simulink model "LKAS"  (R2023b)
settings: Solver=FixedStepDiscrete  StartTime=0.0  StopTime=50  RelTol=1e-3  EnableMultiTasking=on
undefined symbols (not defined in the file): Rec, SDTV
libraries: visionconversions x2, visiongeotforms x2, dspvision x1, slpidlib x1
settings Model: Creator=Aral_Sarrafi  LastModifiedBy=seame-workstation09
settings SolverCC: AlgebraicLoopSolver=TrustRegion  PositivePriorityOrder=on
settings DataIOCC: ReturnWorkspaceOutputs=off
settings OptimizationCC: UseDivisionForNetSlopeComputation=on  GainParamInheritBuiltInType=on  UseFloatMulNetSlope=on  PassReuseOutputArgsAs=Individual arguments  ZeroExternalMemoryAtStartup=off  ZeroInternalMemoryAtStartup=off  NoFixptDivByZeroProtection=on  EfficientFloat2IntCast=on  LifeSpan=1  MaxStackSize=64  OptimizeBlockOrder=speed  OptimizationPriority=Speed  LabelGuidedReuse=on  MultiThreadedLoops=on  EfficientTunableParamExpr=on
settings DebuggingCC: ParameterTunabilityLossMsg=error  UnconnectedInputMsg=warning  UnconnectedOutputMsg=warning  UnconnectedLineMsg=warning  ArithmeticOperatorsInVariantConditions=warning
settings HardwareCC: ProdBitPerPointer=32  ProdBitPerSizeT=32  ProdBitPerPtrDiffT=32  ProdLargestAtomicInteger=Long  ProdLargestAtomicFloat=Double  ProdWordSize=32  ProdLongLongMode=on  ProdHWDeviceType=ARM Compatible->ARM Cortex  TargetBitPerLong=64  TargetBitPerPointer=64  TargetBitPerSizeT=64  TargetBitPerPtrDiffT=64  TargetLongLongMode=on  TargetIntDivRoundTo=Zero  TargetEndianess=LittleEndian  TargetWordSize=64  TargetHWDeviceType=MATLAB Host  ProdEqTarget=off
settings ModelReferenceCC: EnableRefExpFcnMdlSchedulingChecks=on
settings SFSimCC: SimUseLocalCustomCode=off  SimGenImportedTypeDefs=on  MATLABDynamicMemAllocThreshold=0  CustomCodeUndefinedFunction=UseInterfaceOnly  SimTargetLang=C++
settings RTWCC: Description=Embedded Coder  SystemTargetFile=ert.tlc  HardwareBoard=Raspberry Pi  TLCOptions="-aInlineSetEventsForThisBaseRateFcn=TLC_TRUE -aSuppressMultiTaskScheduler=TLC_FALSE  -aRateBasedStepFcn=0"  PackageGeneratedCodeAndArtifacts=on  TemplateMakefile=ert_default_tmf  RTWUseLocalCustomCode=off  TargetLang=C++
settings CodeAppCC: ForceParamTrailComments=on  IgnoreCustomStorageClasses=off  MaxIdLength=63  OperatorAnnotations=on  SimulinkDataObjDesc=on  SFDataObjDesc=on  CustomSymbolStrGlobalVar=rt$N$M  CustomSymbolStrType=$N$M  CustomSymbolStrFcn=$N$M$F  CustomSymbolStrMacro=$N$M  InsertBlockDesc=on
settings ERTTargetCC: IncludeMdlTerminateFcn=off  CombineSignalStateStructs=on  SupportAbsoluteTime=off  SupportComplex=off  SupportNonInlinedSFcns=on  SupportVariableSizeSignals=on  OptimizeReductions=on  ExtModeTransport=2  ExtModeStaticAlloc=on  ExtModeMexFile=ext_xcp  ExtModeIntrfLevel=Level2 - Open  RootIOFormat=Structure reference  ERTFilePackagingFormat=CompactWithDataFile

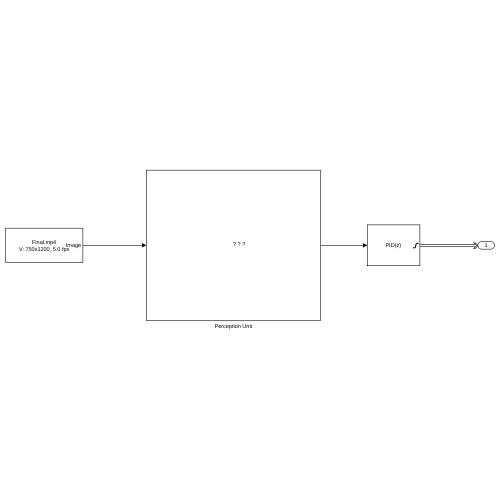
[thumbnail: Simulink's stored preview of the top-level diagram]
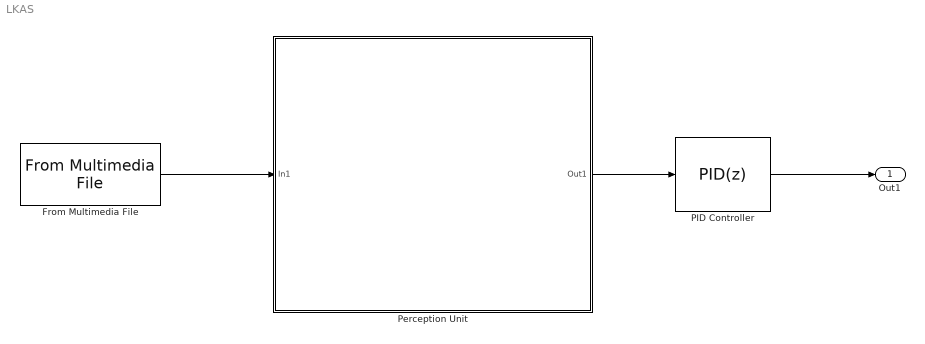
== system LKAS ==
  From Multimedia File : dspvision/From Multimedia File  inputFilename=/home/seame-workstation09/DES_Adaptive-Application/Perception/Final.mp4  readRange=[1 Inf]  loop=on  numPlays=inf  outputStreams=Video only  videoDataType=single  audioDataType=int16  inheritSampleTime=on  userDefinedSampleTime=1/30  noAudioOutput=off  isIntensityVideo=off  fourcc=RGB  colorVideoFormat=One multidimensional signal  outputEOF=off  dataOrg=Column-major  audioFrameSize=1024  computeAudioFrameSize=off  outSamplingMode=Sample based
      settings: LibrarySourceBlock=visionsources/From Multimedia File
  PID Controller : slpidlib/PID Controller  Controller=PID  Form=Parallel  TimeDomain=Discrete-time  UseExternalTs=off  SampleTime=-1  IntegratorMethod=Forward Euler  FilterMethod=Forward Euler  ControllerParametersSource=internal  P=0.015  I=0.02  UseKiTs=off  D=0.012  N=100  UseFilter=on  TunerSelectOption=Transfer Function Based (PID Tuner App)  InitialConditionSource=internal  InitialConditionForIntegrator=0  InitialConditionForFilter=0  DifferentiatorICPrevScaledInput=0  ExternalReset=none  TrackingMode=off  Kt=1  LimitOutput=on  SatLimitsSource=internal  UpperSaturationLimit=pi/2  LowerSaturationLimit=-pi/2  LinearizeAsGain=off  AntiWindupMode=back-calculation  Kb=1  LimitIntegrator=off  UpperIntegratorSaturationLimit=inf  LowerIntegratorSaturationLimit=-inf  POutMin=[]  POutMax=[]  IOutMin=[]  IOutMax=[]  DOutMin=[]  DOutMax=[]  NOutMin=[]  NOutMax=[]  SumOutMin=[]  SumOutMax=[]  SaturationOutMin=[]  SaturationOutMax=[]  PParamMin=[]  PParamMax=[]  IParamMin=[]  IParamMax=[]  DParamMin=[]  DParamMax=[]  NParamMin=[]  NParamMax=[]  KbParamMin=[]  KbParamMax=[]  KtParamMin=[]  KtParamMax=[]  KbOutMin=[]  KbOutMax=[]  KtOutMin=[]  KtOutMax=[]  IntegratorOutMin=[]  IntegratorOutMax=[]  FilterOutMin=[]  FilterOutMax=[]  SumI1OutMin=[]  SumI1OutMax=[]  SumI2OutMin=[]  SumI2OutMax=[]  SumI3OutMin=[]  SumI3OutMax=[]  SumI4OutMin=[]  SumI4OutMax=[]  SumDOutMin=[]  SumDOutMax=[]  DifferentiatorOutMin=[]  DifferentiatorOutMax=[]  FilterDiffOutCoefMin=[]  FilterDiffOutCoefMax=[]  ReciprocalOutMin=[]  ReciprocalOutMax=[]  SumDenOutMin=[]  SumDenOutMax=[]  SumNumOutMin=[]  SumNumOutMax=[]  DivideOutMin=[]  DivideOutMax=[]  UdiffTsProdOutMin=[]  UdiffTsProdOutMax=[]  NTsProdOutMin=[]  NTsProdOutMax=[]  UintegralTsProdOutMin=[]  UintegralTsProdOutMax=[]  UngainTsProdOutMin=[]  UngainTsProdOutMax=[]  ClampingZeroOutDataTypeStr=Inherit: Inherit via back propagation  ClampingZeroOutMin=[]  ClampingZeroOutMax=[]  FilterDenConstantOutDataTypeStr=Inherit: Inherit via back propagation  FilterDenConstantOutMin=[]  FilterDenConstantOutMax=[]  PCopyOutDataTypeStr=Inherit: Inherit via back propagation  PCopyOutMin=[]  PCopyOutMax=[]  NCopyOutDataTypeStr=Inherit: Inherit via back propagation  NCopyOutMin=[]  NCopyOutMax=[]  IntegratorContinuousStateAttributes=''  IntegratorStateMustResolveToSignalObject=off  IntegratorRTWStateStorageClass=Auto  FilterContinuousStateAttributes=''  FilterStateMustResolveToSignalObject=off  FilterRTWStateStorageClass=Auto  ParallelPVariant=InternalParameters  IdealPVariant=Disabled  IVariant=InternalParameters  DVariant=InternalParameters  IntegratorVariant=Discrete  SatVariant=Enabled  AWVariant=BackCalculation  PCopyVariant=Disabled  TRVariant=Disabled  FdbkBlocksVariant=Forward  IdealPFdbkVariant=Disabled  SatFdbkVariant=Disabled  DerivativeFilterVariant=ForwardEulerFilter  NVariant=InternalParameters  NCopyVariant=Disabled  FilterICVariant=InternalICsFilter  IntegratorICVariant=InternalICs  ExternalResetVariant=Disabled  TRSumVariant=Passthrough  SumFdbkVariant=Disabled  SumVariant=Sum_PID  TsampFilterVariant=InternalTs  TsampNgainVariant=Passthrough  TsampIntegralVariant=Disabled_SignalSpec  ExternalSaturationOutDataTypeStr=Inherit: Same as second input
  Perception Unit : Subsystem
      mask Display: image('computer-vision.jpg');
  Out1 : Outport
  wires:
  Perception Unit/1(Out1) -> PID Controller/1
  From Multimedia File/1 -> Perception Unit/1(In1)
  PID Controller/1 -> Out1/1

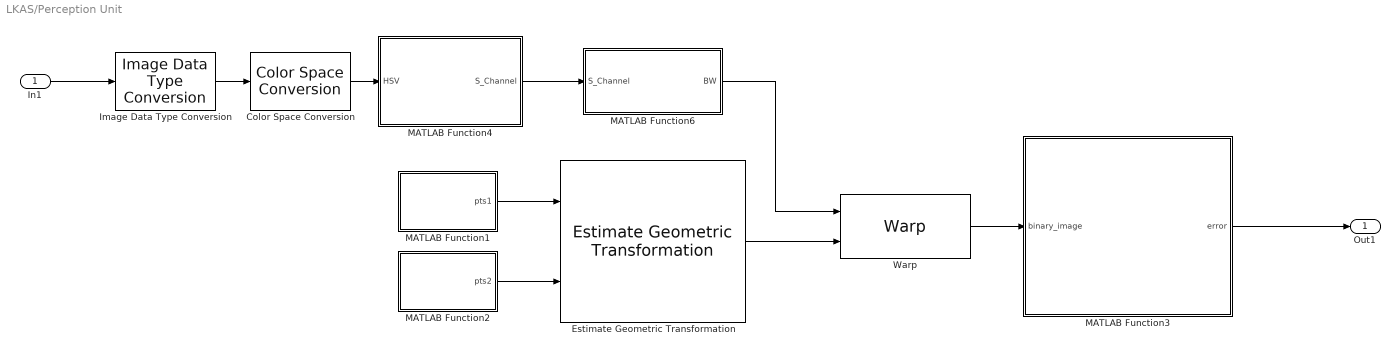
== system LKAS/Perception Unit ==
  In1 : Inport
  Color Space Conversion : visionconversions/Color Space  Conversion  conversion=Obsolete  conversionActive=R'G'B' to HSV  wp_str=D65  rec=Rec. 601 (SDTV)  sys=1125/60/2:1  imagePorts=One multidimensional signal
  Estimate Geometric Transformation : visiongeotforms/Estimate Geometric Transformation  tformType=Projective  isRandomSampling=on  algMethod=Random Sample Consensus (RANSAC)  distanceAlg=2.5  distanceGeo=2.5  numMethod=Specified value  sampleNum=500  desiredConfidence=99  maxSampleNum=1000  isStopSampling=off  percentStop=75  isRefineTForm=off  isReleaseMode=on  isOutputInlier=off  outDT4IntInput=Obsolete10a  outDT4IntInputActive=Single  isVarSizeAllowed=on
  Image Data Type Conversion : visionconversions/Image Data Type Conversion  outDT=double  isSigned=on  wordLen=16  numFracBits=0
  MATLAB Function1 : MATLAB Function  TreatAsAtomicUnit=on
  MATLAB Function2 : MATLAB Function  TreatAsAtomicUnit=on
  MATLAB Function3 : MATLAB Function  TreatAsAtomicUnit=on
  MATLAB Function4 : MATLAB Function  TreatAsAtomicUnit=on
  MATLAB Function6 : MATLAB Function  TreatAsAtomicUnit=on
  Warp : visiongeotforms/Warp  TransformMatrixSource=Input port  TransformMatrix=eye( 3 )  InterpolationMethod=Bilinear  BackgroundFillValue=0  OutputImagePositionSource=Same as input image  OutputImagePosition=[ 1, 1, 512, 512 ]  ROIInputPort=off  ROIValidityOutputPort=off  SimulateUsing=Interpreted execution
  Out1 : Outport  VectorParamsAs1DForOutWhenUnconnected=off
  wires:
  MATLAB Function1/1(pts1) -> Estimate Geometric Transformation/1
  Estimate Geometric Transformation/1 -> Warp/2
  MATLAB Function2/1(pts2) -> Estimate Geometric Transformation/2
  MATLAB Function3/1(error) -> Out1/1
  Color Space Conversion/1 -> MATLAB Function4/1(HSV)
  In1/1 -> Image Data Type Conversion/1
  Image Data Type Conversion/1 -> Color Space Conversion/1
  MATLAB Function6/1(BW) -> Warp/1
  MATLAB Function4/1(S_Channel) -> MATLAB Function6/1(S_Channel)
  Warp/1 -> MATLAB Function3/1(binary_image)

== matlab function LKAS/Perception Unit/MATLAB Function1 ==
  data: pts1 output
function pts1 = getpts1()

pts1 = [519 411
        675 411
        113 587
        1049 587];

end

== matlab function LKAS/Perception Unit/MATLAB Function2 ==
  data: pts2 output
function pts2 = getpts2()

h = 750; 
w = 1200;

pts2 = [450 0
        w-450 0
        450 h
        w-450 h];

end

== matlab function LKAS/Perception Unit/MATLAB Function3 ==
  data: binary_image input; error output
function error   = Lane_Detection(binary_image)

h = size(binary_image,1);
w = size(binary_image,2);

mid_h = h/2;

base = sum(binary_image(mid_h:end,:)); % 이미지 하단 ~ mid_h까지 각 열에 대한 픽셀 합 (sum of pixel value from mid_h to end of the image)


mid_w = w/2;

[~,locs] = findpeaks(base); % peak(값이 큰 열 = 차선)의 index를 locs로 반환 (return peak value from base)
left_base = locs(1); % locs 중 첫번째(가장 왼쪽)을 왼쪽 차선 기본위치로 선정� (first index of locs is considered as left_base)

right_base = locs(locs - left_base > 200); % left_base(왼쪽 차선)에서 최소 200 픽셀 이상 떨어져 있는 index를 right_base로 반환 (indexs 200 pixels after left_base are stored to right_base)
right_base = right_base(end); % 그 중 가장 끝(오른쪽)을 오른쪽 차선 기본위치로 선정 (and the end index of right_base is considered as right_base)

nwindows = 10; % 윈도우 개수 (number of windows)

window_hight = h/nwindows; % 윈도우별 높이(고정) (height of each window)

leftx_current = left_base;
rightx_current = right_base;

margin = 80; % 윈도우 너비 결정 (margin determine width of window)
minpix = 40;

max_points = 100000; % 정적 배열 할당 위한 행(point 개수) 지정 (maximum size of row for static array)

% 슬라이딩 윈도우를 통해 탐색된 차선 픽셀들 담을 list (list for storing pixels which are found
% from sliding window algorithm)
% method1: static
left_lane_index = zeros(max_points, 2);
right_lane_index = zeros(max_points, 2);


[nonzeroy, nonzerox] = find(binary_image); % 흰색 픽셀(차선)의 x, y 좌표 찾음 (found pixel's location which has '1' value(which means white))


rectangle_points = zeros(2 * nwindows,4); % 각 윈도우들의 경계를 저장하기 위한 행렬, 0으로 초기화, 윈도우 개수*2(왼쪽, 오른쪽), 4개의 열(x, y, w, h) (setting array for each widow's boundary)


% static 
count_left = 0; % 몇개의 행(points)이 사용됐는지 추적 위한 count (to count how many points are stored)
count_right = 0;



for i = 0:nwindows-1
    %Loop over the windows to find the nonzero elements in the selected
    %window
        
        % 좌측, 우측 윈도우 사이즈 (size of window)
        win_y_low = h - (i+1)*window_hight;
        win_y_high = h - i*window_hight;
        
        win_xleft_low = leftx_current - margin;
        win_xleft_high = leftx_current + margin;
        
        win_xright_low = rightx_current - margin;
        win_xright_high = rightx_current + margin;
        

        
        rectangle_points(i+1,:) = [win_xleft_low win_y_low 2*margin window_hight]; % rectangle_points 행렬에 좌측 차선 윈도우 경계 저장 ([x, y, w, h]) (store window's boundary to rectangle_points)
        rectangle_points(nwindows + 1 + i,:) = [win_xright_low win_y_low 2*margin window_hight]; % rectangle_points 행렬에 우측 차선 윈도우 경계 저장 ([x, y, w, h])
        

        % 현재 윈도우에서 흰색 픽샐 인덱스 추출 (get pixel index within window)
        good_leftx_indexs = nonzerox((nonzeroy >= win_y_low) & (nonzeroy < win_y_high) & (nonzerox >= win_xleft_low) &  (nonzerox < win_xleft_high)); 
        good_lefty_indexs = nonzeroy((nonzeroy >= win_y_low) & (nonzeroy < win_y_high) & (nonzerox >= win_xleft_low) &  (nonzerox < win_xleft_high));
        
        good_rightx_indexs = nonzerox((nonzeroy >= win_y_low) & (nonzeroy < win_y_high) & (nonzerox >= win_xright_low) &  (nonzerox < win_xright_high));
        good_righty_indexs = nonzeroy((nonzeroy >= win_y_low) & (nonzeroy < win_y_high) & (nonzerox >= win_xright_low) &  (nonzerox < win_xright_high));
        
        % 왼쪽차선, 오른쪽차선 인덱스 list에 추출된 픽셀 인덱스를 각각 추가 (store indeox found from
        % current window to array)
        % method1: static 
        for j = count_left+1:numel(good_leftx_indexs)
            left_lane_index(j, :) = [good_leftx_indexs(j), good_lefty_indexs(j)];
            count_left = count_left + 1;
        end

        for j = count_right+1:numel(good_rightx_indexs)
            right_lane_index(j, :) = [good_rightx_indexs(j), good_righty_indexs(j)];
            count_right = count_right + 1;
        end
        

        % 현재 윈도우에서 찾은 픽셀이 일정 minpix보다 클 경우, x의 평균값(윈도우 내 탐색된 차선 픽셀들의 평균)으로 x_current 값 업데이트 
        % minpix보다 작을 경우 이전 x_current 값으로 그대로 올려서 재탐색
        % (if num of pixels froum current window is bigger than minpix,
        % update x_current)
        if(numel(good_leftx_indexs) > minpix)
            leftx_current = mean(good_leftx_indexs);
            
        end
        
        if(numel(good_rightx_indexs) > minpix)
            rightx_current = mean(good_rightx_indexs);
            
        end
          
end

% static
actual_left_lane_index = left_lane_index(1:count_left, :);
actual_right_lane_index = right_lane_index(1:count_right, :);

% 검출된 차선 픽셀들 이용하여 2차 다항식으로 차선 모델링
% static
p_left = polyfit(actual_left_lane_index(:,2),actual_left_lane_index(:,1),2); % p_left: 왼쪽 다항식의 계수를 나타내는 벡터 
p_right = polyfit(actual_right_lane_index(:,2),actual_right_lane_index(:,1),2); % p_right: 오른쪽 다항식의 계수를 나타내는 벡터



y = 0:1:h; % 0~h 까지 1씩 증가하는 값을 가지는 y벡터 (0,1,2,...,h) 

xleft = polyval(p_left,y); % 피팅된 다항식을 이용해 y값에 대응하는 X 값 계산 (get x value corresponding to y value) 
xright = polyval(p_right,y);

error = mid_w - (xleft(end)+xright(end))/2;


end

== matlab function LKAS/Perception Unit/MATLAB Function6 ==
  data: BW output; S_Channel input
function BW = mask(S_Channel)
S_th = 0.75;

BW = S_Channel > S_th;

end

== matlab function LKAS/Perception Unit/MATLAB Function4 ==
  data: S_Channel output; HSV input
function S_Channel = get_SChannel(HSV)

S_Channel = HSV(:,:,2);

end
